simulink model "2_Link_Manipulator(PID)"  (R2024a)
settings: Solver=ode45  StartTime=0.0  StopTime=10  RelTol=1e-3
model workspace (MAT data in the model file):
  input1 = Simulink.Parameter
  input1.Complexity = 'real'
  input1.Dimensions = [0 0]
  input1.DataType = 'auto'
settings Model: Creator=Aryan Shrivastava  LastModifiedBy=Aryan Shrivastava
settings SolverCC: MaxConsecutiveMinStep=5

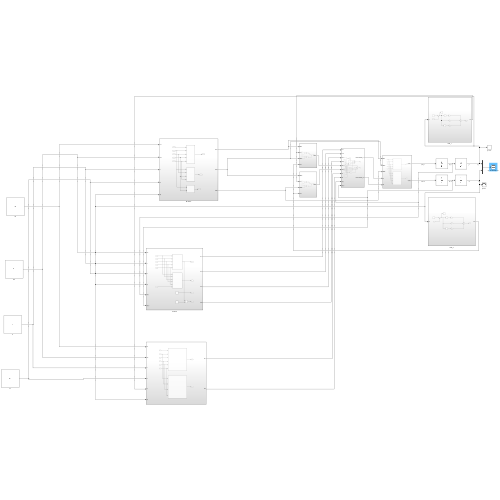
[thumbnail: Simulink's stored preview of the top-level diagram]
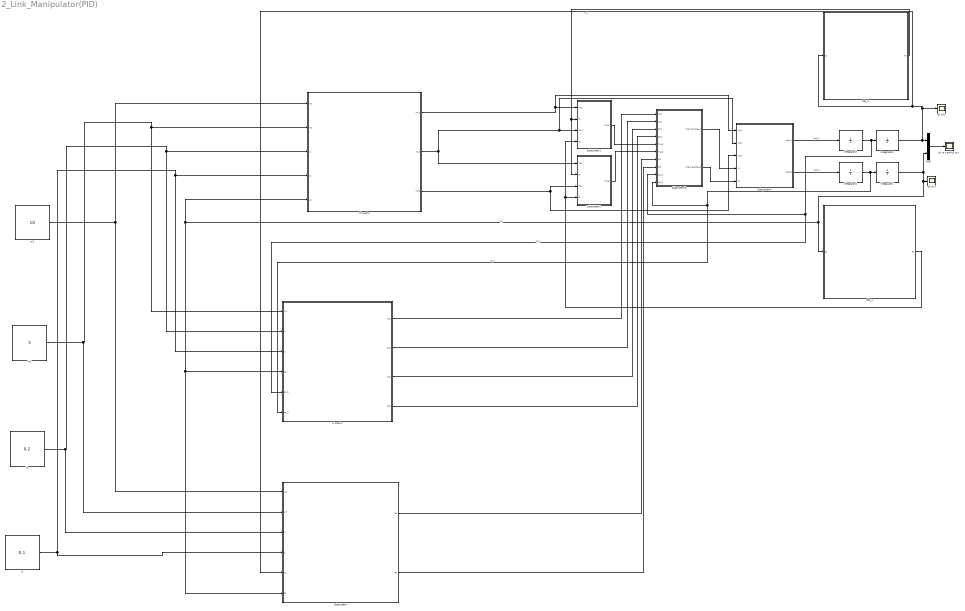
== system 2_Link_Manipulator(PID) ==
  C matrix : Subsystem
  Integrator1 : Integrator  InitialCondition=0.1
  Integrator2 : Integrator
  Integrator3 : Integrator  InitialCondition=0.1
  Integrator4 : Integrator
  M matrix : Subsystem
  Mux : Mux  Inputs=2
  PID_1 : Subsystem
  PID_2 : Subsystem
  Subsystem : Subsystem
  Subsystem1 : Subsystem
  Subsystem2 : Subsystem
  Subsystem3 : Subsystem
  Subsystem4 : Subsystem
  l1 : Constant  Value=0.2
  l2 : Constant  Value=0.1
  m1 : Constant  Value=10
  m2 : Constant  Value=5
  q1 vs t : Scope
  q1 vs t and q2 vs t : Scope
  q2 vs t : Scope
  wires:
  Subsystem2/1(TAU2) -> Subsystem3/6(TAU2)
  Subsystem1/1(TAU1) -> Subsystem3/5(TAU1)
  Subsystem3/1(Intermediate_1) -> Subsystem4/4(I1)
  Subsystem3/2(Intermediate_2) -> Subsystem4/5(I2)
  Integrator2/1 -> Subsystem3/9(qd_1), C matrix/5(qd_1), Integrator3/1  "qd_1"
  Integrator4/1 -> Subsystem3/10(qd_2), C matrix/6(qd_2), Integrator1/1  "qd_2"
  Subsystem4/2(qdd_2) -> Integrator4/1  "qdd_2"
  Subsystem4/1(qdd_1) -> Integrator2/1  "qdd_1"
  Mux/1 -> q1 vs t and q2 vs t/1
  m1/1 -> Subsystem/1(m1), M matrix/1(m1)
  m2/1 -> Subsystem/2(m2), C matrix/1(m2), M matrix/2(m2)
  l1/1 -> Subsystem/3(l1), C matrix/2(l1), M matrix/3(l1)
  l2/1 -> Subsystem/4(l2), C matrix/3(l2), M matrix/4(l2)
  M matrix/1(M11) -> Subsystem4/1(M11), Subsystem1/1(M11)
  M matrix/2(M12) -> Subsystem4/2(M12), Subsystem1/3(M12), Subsystem2/1(M12)
  M matrix/3(M22) -> Subsystem2/3(M22), Subsystem4/3(M22)
  PID_1/1(F1) -> Subsystem2/2(F1), Subsystem1/2(F1)
  PID_2/1(F2) -> Subsystem1/4(F2), Subsystem2/4(F2)
  C matrix/1(C11) -> Subsystem3/1(C11)
  C matrix/2(C12) -> Subsystem3/2(C12)
  C matrix/3(C21) -> Subsystem3/3(C21)
  C matrix/4(C22) -> Subsystem3/4(C22)
  Subsystem/1(G1) -> Subsystem3/7(G1)
  Subsystem/2(G2) -> Subsystem3/8(G2)
  Integrator3/1 -> Mux/1, q1 vs t/1, Subsystem/5(q1), PID_1/1(q1)  "q_1"
  Integrator1/1 -> Subsystem/6(q2), C matrix/4(q2), M matrix/5(q2), PID_2/1(q2), q2 vs t/1, Mux/2  "q_2"

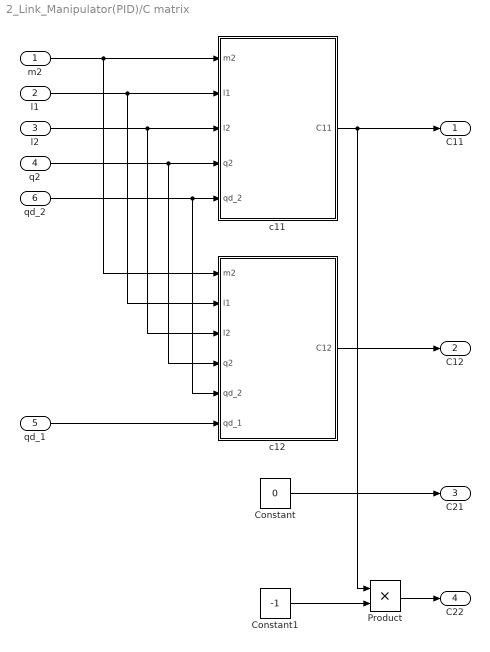
== system 2_Link_Manipulator(PID)/C matrix ==
  m2 : Inport
  l1 : Inport  Port=2
  l2 : Inport  Port=3
  q2 : Inport  Port=4
  qd_1 : Inport  Port=5
  qd_2 : Inport  Port=6
  Constant : Constant  Value=0
  Constant1 : Constant  Value=-1
  Product : Product
  c11 : Subsystem
  c12 : Subsystem
  C11 : Outport
  C12 : Outport  Port=2
  C21 : Outport  Port=3
  C22 : Outport  Port=4
  wires:
  Constant/1 -> C21/1
  c11/1(C11) -> Product/1, C11/1
  Constant1/1 -> Product/2
  m2/1 -> c12/1(m2), c11/1(m2)
  l1/1 -> c12/2(l1), c11/2(l1)
  l2/1 -> c12/3(l2), c11/3(l2)
  q2/1 -> c12/4(q2), c11/4(q2)
  qd_2/1 -> c12/5(qd_2), c11/5(qd_2)
  qd_1/1 -> c12/6(qd_1)
  c12/1(C12) -> C12/1
  Product/1 -> C22/1

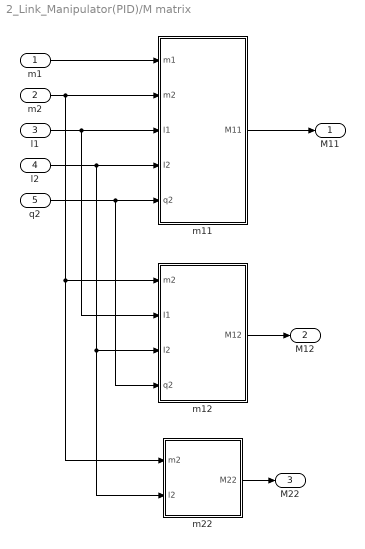
== system 2_Link_Manipulator(PID)/M matrix ==
  m1 : Inport
  m2 : Inport  Port=2
  l1 : Inport  Port=3
  l2 : Inport  Port=4
  q2 : Inport  Port=5
  m11 : Subsystem
  m12 : Subsystem
  m22 : Subsystem
  M11 : Outport
  M12 : Outport  Port=2
  M22 : Outport  Port=3
  wires:
  m1/1 -> m11/1(m1)
  m2/1 -> m22/1(m2), m12/1(m2), m11/2(m2)
  l1/1 -> m12/2(I1), m11/3(l1)
  l2/1 -> m22/2(l2), m12/3(I2), m11/4(I2)
  q2/1 -> m12/4(q2), m11/5(q2)
  m11/1(M11) -> M11/1
  m12/1(M12) -> M12/1
  m22/1(M22) -> M22/1

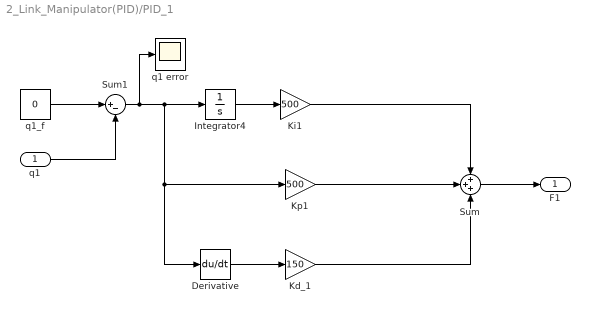
== system 2_Link_Manipulator(PID)/PID_1 ==
  q1 : Inport
  Derivative : Derivative
  Integrator4 : Integrator  InitialCondition=0.1
  Kd_1 : Gain  Gain=150
  Ki1 : Gain  Gain=500
  Kp1 : Gain  Gain=500
  Sum : Sum  Inputs=+++
  Sum1 : Sum  Inputs=|+-
  q1 error : Scope
  q1_f : Constant  Value=0
  F1 : Outport
  wires:
  Ki1/1 -> Sum/1
  Kd_1/1 -> Sum/3
  Sum/1 -> F1/1
  Kp1/1 -> Sum/2
  Integrator4/1 -> Ki1/1
  Sum1/1 -> q1 error/1, Integrator4/1, Derivative/1, Kp1/1
  q1/1 -> Sum1/2
  q1_f/1 -> Sum1/1
  Derivative/1 -> Kd_1/1

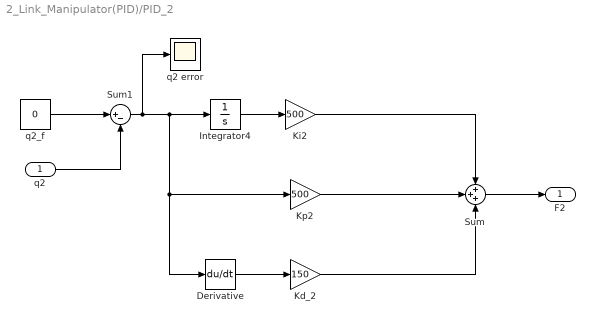
== system 2_Link_Manipulator(PID)/PID_2 ==
  q2 : Inport
  Derivative : Derivative
  Integrator4 : Integrator
  Kd_2 : Gain  Gain=150
  Ki2 : Gain  Gain=500
  Kp2 : Gain  Gain=500
  Sum : Sum  Inputs=+++
  Sum1 : Sum  Inputs=|+-
  q2 error : Scope
  q2_f : Constant  Value=0
  F2 : Outport
  wires:
  Ki2/1 -> Sum/1
  Kd_2/1 -> Sum/3
  Sum/1 -> F2/1
  Kp2/1 -> Sum/2
  Integrator4/1 -> Ki2/1
  Sum1/1 -> q2 error/1, Integrator4/1, Derivative/1, Kp2/1
  q2/1 -> Sum1/2
  q2_f/1 -> Sum1/1
  Derivative/1 -> Kd_2/1

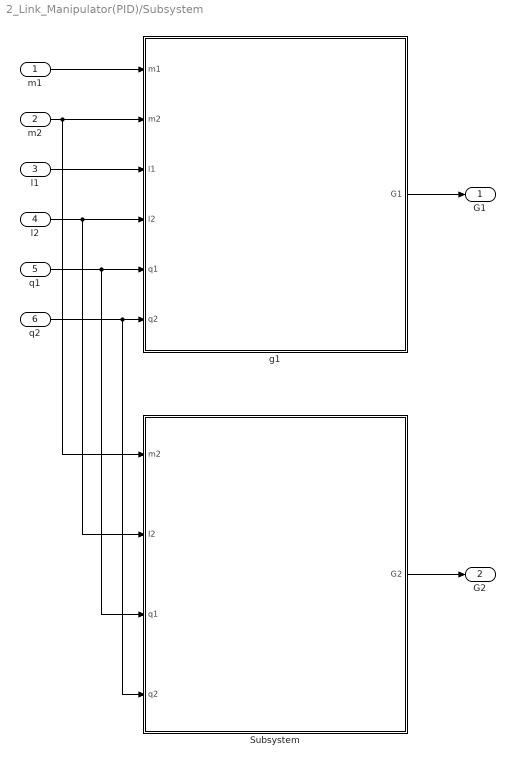
== system 2_Link_Manipulator(PID)/Subsystem ==
  m1 : Inport
  m2 : Inport  Port=2
  l1 : Inport  Port=3
  l2 : Inport  Port=4
  q1 : Inport  Port=5
  q2 : Inport  Port=6
  Subsystem : Subsystem
  g1 : Subsystem
  G1 : Outport
  G2 : Outport  Port=2
  wires:
  m2/1 -> g1/2(m2), Subsystem/1(m2)
  m1/1 -> g1/1(m1)
  l1/1 -> g1/3(l1)
  l2/1 -> Subsystem/2(I2), g1/4(l2)
  q1/1 -> g1/5(q1), Subsystem/3(q1)
  q2/1 -> Subsystem/4(q2), g1/6(q2)
  g1/1(G1) -> G1/1
  Subsystem/1(G2) -> G2/1

== system 2_Link_Manipulator(PID)/Subsystem1 ==
  M11 : Inport
  F1 : Inport  Port=2
  M12 : Inport  Port=3
  F2 : Inport  Port=4
  Product : Product
  Product1 : Product
  Sum : Sum  Inputs=|++
  TAU1 : Outport
  wires:
  M11/1 -> Product/1
  F1/1 -> Product/2
  M12/1 -> Product1/1
  F2/1 -> Product1/2
  Product/1 -> Sum/1
  Product1/1 -> Sum/2
  Sum/1 -> TAU1/1

== system 2_Link_Manipulator(PID)/Subsystem2 ==
  M12 : Inport
  F1 : Inport  Port=2
  M22 : Inport  Port=3
  F2 : Inport  Port=4
  Product : Product
  Product1 : Product
  Sum : Sum  Inputs=|++
  TAU2 : Outport
  wires:
  Product1/1 -> Sum/2
  F1/1 -> Product/2
  F2/1 -> Product1/2
  M12/1 -> Product/1
  Product/1 -> Sum/1
  M22/1 -> Product1/1
  Sum/1 -> TAU2/1

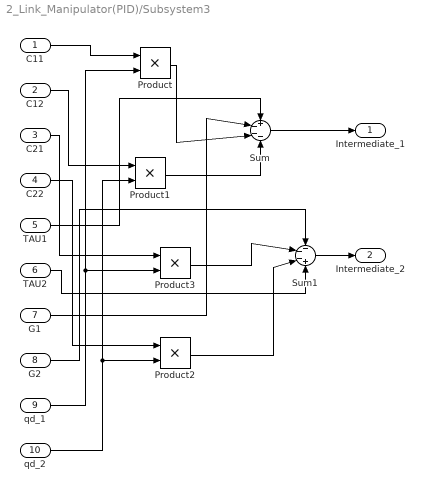
== system 2_Link_Manipulator(PID)/Subsystem3 ==
  C11 : Inport
  C12 : Inport  Port=2
  C21 : Inport  Port=3
  C22 : Inport  Port=4
  TAU1 : Inport  Port=5
  TAU2 : Inport  Port=6
  G1 : Inport  Port=7
  G2 : Inport  Port=8
  qd_1 : Inport  Port=9
  qd_2 : Inport  Port=10
  Product{,1..3} (4 alike) : Product
  Sum : Sum  Inputs=+---
  Sum1 : Sum  Inputs=---+
  Intermediate_1 : Outport
  Intermediate_2 : Outport  Port=2
  wires:
  G1/1 -> Sum/2
  TAU1/1 -> Sum/1
  C11/1 -> Product/1
  qd_1/1 -> Product3/2, Product/2
  Product/1 -> Sum/3
  C12/1 -> Product1/1
  qd_2/1 -> Product2/2, Product1/2
  Product1/1 -> Sum/4
  Sum/1 -> Intermediate_1/1
  C21/1 -> Product3/1
  C22/1 -> Product2/1
  TAU2/1 -> Sum1/4
  Product3/1 -> Sum1/2
  Product2/1 -> Sum1/3
  G2/1 -> Sum1/1
  Sum1/1 -> Intermediate_2/1

== system 2_Link_Manipulator(PID)/Subsystem4 ==
  M11 : Inport
  M12 : Inport  Port=2
  M22 : Inport  Port=3
  I1 : Inport  Port=4
  I2 : Inport  Port=5
  Subsystem : Subsystem
  Subsystem1 : Subsystem
  qdd_1 : Outport
  qdd_2 : Outport  Port=2
  wires:
  M12/1 -> Subsystem1/2(M12), Subsystem/2(M12)
  M11/1 -> Subsystem/1(M11), Subsystem1/1(M11)
  M22/1 -> Subsystem1/3(M22), Subsystem/3(M22)
  I1/1 -> Subsystem1/4(I1), Subsystem/4(I1)
  I2/1 -> Subsystem1/5(I2), Subsystem/5(I2)
  Subsystem/1(qdd_1) -> qdd_1/1
  Subsystem1/1(qdd_2) -> qdd_2/1

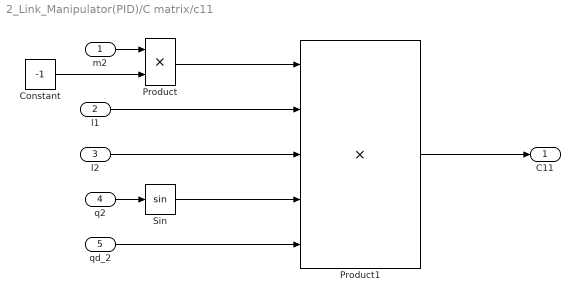
== system 2_Link_Manipulator(PID)/C matrix/c11 ==
  m2 : Inport
  l1 : Inport  Port=2
  l2 : Inport  Port=3
  q2 : Inport  Port=4
  qd_2 : Inport  Port=5
  Constant : Constant  Value=-1
  Product : Product
  Product1 : Product  Inputs=5
  Sin : Trigonometry
  C11 : Outport
  wires:
  q2/1 -> Sin/1
  m2/1 -> Product/1
  Constant/1 -> Product/2
  qd_2/1 -> Product1/5
  Sin/1 -> Product1/4
  l2/1 -> Product1/3
  l1/1 -> Product1/2
  Product/1 -> Product1/1
  Product1/1 -> C11/1

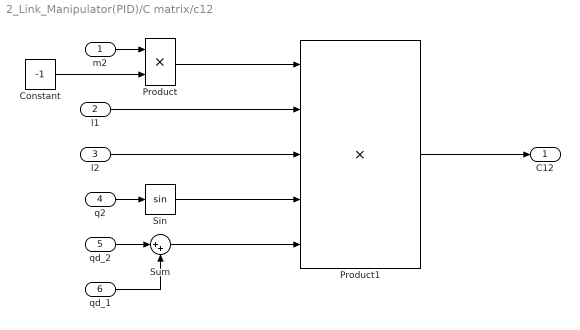
== system 2_Link_Manipulator(PID)/C matrix/c12 ==
  m2 : Inport
  l1 : Inport  Port=2
  l2 : Inport  Port=3
  q2 : Inport  Port=4
  qd_2 : Inport  Port=5
  qd_1 : Inport  Port=6
  Constant : Constant  Value=-1
  Product : Product
  Product1 : Product  Inputs=5
  Sin : Trigonometry
  Sum : Sum  Inputs=|++
  C12 : Outport
  wires:
  q2/1 -> Sin/1
  m2/1 -> Product/1
  Constant/1 -> Product/2
  Sin/1 -> Product1/4
  l2/1 -> Product1/3
  l1/1 -> Product1/2
  Product/1 -> Product1/1
  Product1/1 -> C12/1
  qd_2/1 -> Sum/1
  qd_1/1 -> Sum/2
  Sum/1 -> Product1/5

== system 2_Link_Manipulator(PID)/M matrix/m11 ==
  m1 : Inport
  m2 : Inport  Port=2
  l1 : Inport  Port=3
  I2 : Inport  Port=4
  q2 : Inport  Port=5
  Subsystem : Subsystem
  Subsystem1 : Subsystem
  Sum : Sum  Inputs=|++
  M11 : Outport
  wires:
  m1/1 -> Subsystem/1(m1)
  m2/1 -> Subsystem1/1(m2), Subsystem/2(m2)
  l1/1 -> Subsystem1/2(l1), Subsystem/3(I1)
  I2/1 -> Subsystem1/3(l2)
  q2/1 -> Subsystem1/4(q2)
  Subsystem/1(m11_1) -> Sum/1
  Subsystem1/1(m11_2) -> Sum/2
  Sum/1 -> M11/1

== system 2_Link_Manipulator(PID)/M matrix/m12 ==
  m2 : Inport
  I1 : Inport  Port=2
  I2 : Inport  Port=3
  q2 : Inport  Port=4
  Cos : Trigonometry  Operator=cos
  Product : Product  Inputs=3
  Product1 : Product
  Sum : Sum  Inputs=|++
  M12 : Outport
  wires:
  m2/1 -> Product/1
  I2/1 -> Product/2, Sum/1
  q2/1 -> Cos/1
  I1/1 -> Product1/1
  Product1/1 -> Sum/2
  Sum/1 -> Product/3
  Product/1 -> M12/1
  Cos/1 -> Product1/2  "cos (q2)"

== system 2_Link_Manipulator(PID)/M matrix/m22 ==
  m2 : Inport
  l2 : Inport  Port=2
  Product : Product
  Square : Math  Operator=square
  M22 : Outport
  wires:
  m2/1 -> Product/1
  l2/1 -> Square/1
  Square/1 -> Product/2
  Product/1 -> M22/1

== system 2_Link_Manipulator(PID)/Subsystem/Subsystem ==
  m2 : Inport
  I2 : Inport  Port=2
  q1 : Inport  Port=3
  q2 : Inport  Port=4
  Constant : Constant  Value=9.81
  Cos : Trigonometry  Operator=cos
  Product : Product  Inputs=4
  Sum : Sum  Inputs=|++
  G2 : Outport
  wires:
  Sum/1 -> Cos/1
  q1/1 -> Sum/1
  q2/1 -> Sum/2
  I2/1 -> Product/2
  m2/1 -> Product/1
  Cos/1 -> Product/3
  Product/1 -> G2/1
  Constant/1 -> Product/4

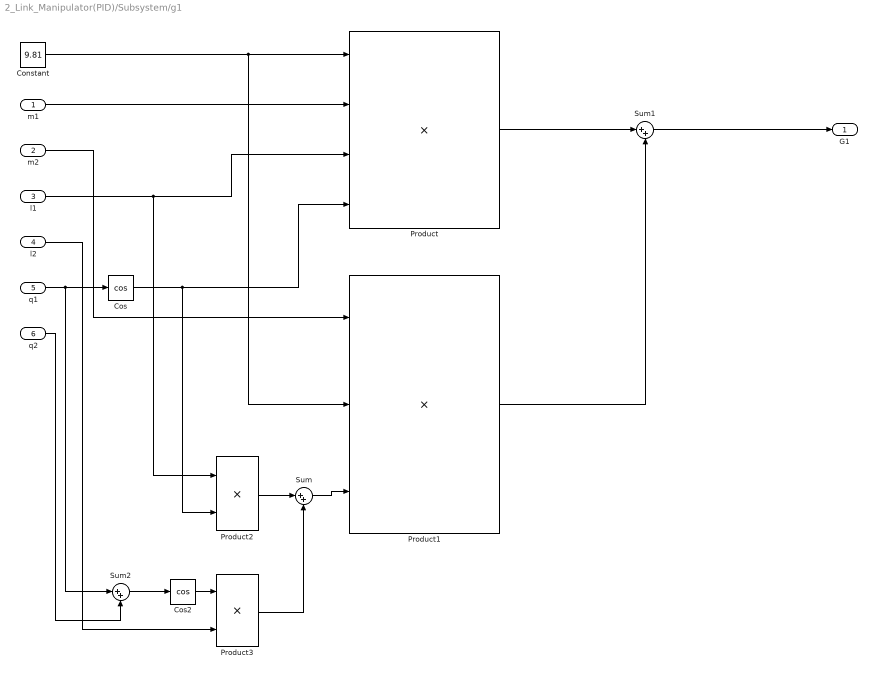
== system 2_Link_Manipulator(PID)/Subsystem/g1 ==
  m1 : Inport
  m2 : Inport  Port=2
  l1 : Inport  Port=3
  l2 : Inport  Port=4
  q1 : Inport  Port=5
  q2 : Inport  Port=6
  Constant : Constant  Value=9.81
  Cos : Trigonometry  Operator=cos
  Cos2 : Trigonometry  Operator=cos
  Product : Product  Inputs=4
  Product1 : Product  Inputs=3
  Product2 : Product
  Product3 : Product
  Sum : Sum  Inputs=|++
  Sum1 : Sum  Inputs=|++
  Sum2 : Sum  Inputs=|++
  G1 : Outport
  wires:
  Cos2/1 -> Product3/1
  m2/1 -> Product1/1
  Sum2/1 -> Cos2/1
  Sum/1 -> Product1/3
  Product1/1 -> Sum1/2
  l1/1 -> Product/3, Product2/1
  q1/1 -> Sum2/1, Cos/1
  l2/1 -> Product3/2
  m1/1 -> Product/2
  Product/1 -> Sum1/1
  Cos/1 -> Product/4, Product2/2
  Product2/1 -> Sum/1
  Product3/1 -> Sum/2
  Constant/1 -> Product1/2, Product/1
  q2/1 -> Sum2/2
  Sum1/1 -> G1/1

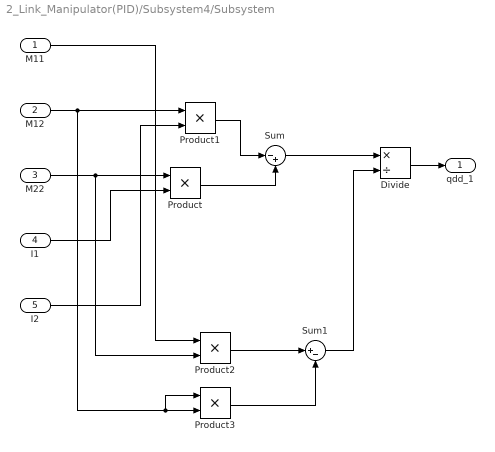
== system 2_Link_Manipulator(PID)/Subsystem4/Subsystem ==
  M11 : Inport
  M12 : Inport  Port=2
  M22 : Inport  Port=3
  I1 : Inport  Port=4
  I2 : Inport  Port=5
  Divide : Product  Inputs=*/
  Product{,1..3} (4 alike) : Product
  Sum : Sum  Inputs=|-+
  Sum1 : Sum  Inputs=|+-
  qdd_1 : Outport
  wires:
  Product1/1 -> Sum/1
  Product/1 -> Sum/2
  Sum1/1 -> Divide/2
  Product3/1 -> Sum1/2
  Product2/1 -> Sum1/1
  I1/1 -> Product/2
  Divide/1 -> qdd_1/1
  M12/1 -> Product3/1, Product3/2, Product1/1
  I2/1 -> Product1/2
  M22/1 -> Product2/2, Product/1
  M11/1 -> Product2/1
  Sum/1 -> Divide/1

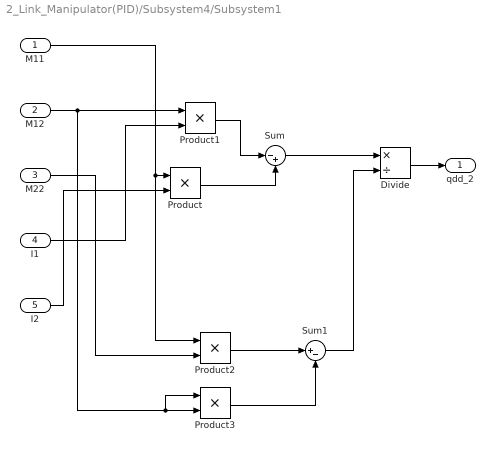
== system 2_Link_Manipulator(PID)/Subsystem4/Subsystem1 ==
  M11 : Inport
  M12 : Inport  Port=2
  M22 : Inport  Port=3
  I1 : Inport  Port=4
  I2 : Inport  Port=5
  Divide : Product  Inputs=*/
  Product{,1..3} (4 alike) : Product
  Sum : Sum  Inputs=|-+
  Sum1 : Sum  Inputs=|+-
  qdd_2 : Outport
  wires:
  Product1/1 -> Sum/1
  Product/1 -> Sum/2
  Sum1/1 -> Divide/2
  Product3/1 -> Sum1/2
  Product2/1 -> Sum1/1
  I1/1 -> Product1/2
  Divide/1 -> qdd_2/1
  M12/1 -> Product3/1, Product3/2, Product1/1
  M22/1 -> Product2/2
  M11/1 -> Product/1, Product2/1
  Sum/1 -> Divide/1
  I2/1 -> Product/2

== system 2_Link_Manipulator(PID)/M matrix/m11/Subsystem ==
  m1 : Inport
  m2 : Inport  Port=2
  I1 : Inport  Port=3
  Product : Product
  Product1 : Product
  Sum : Sum  Inputs=|++
  m11_1 : Outport
  wires:
  Product1/1 -> Product/2
  m1/1 -> Sum/1
  I1/1 -> Product1/2, Product1/1
  m2/1 -> Sum/2
  Sum/1 -> Product/1
  Product/1 -> m11_1/1

== system 2_Link_Manipulator(PID)/M matrix/m11/Subsystem1 ==
  m2 : Inport
  l1 : Inport  Port=2
  l2 : Inport  Port=3
  q2 : Inport  Port=4
  Constant : Constant  Value=2
  Cos : Trigonometry  Operator=cos
  Product : Product  Inputs=3
  Product1 : Product  Inputs=3
  Sum : Sum  Inputs=|++
  m11_2 : Outport
  wires:
  m2/1 -> Product/1
  l2/1 -> Product/2, Sum/1
  q2/1 -> Cos/1
  l1/1 -> Product1/1
  Constant/1 -> Product1/2
  Cos/1 -> Product1/3
  Product1/1 -> Sum/2
  Sum/1 -> Product/3
  Product/1 -> m11_2/1
